simulink model "msgex1_data_vs_event_vs_msg"  (R2018a)
settings: Solver=FixedStepDiscrete  StartTime=0.0  StopTime=10.0  FixedStep=1  RelTol=1e-3  EnableMultiTasking=on
undefined symbols (not defined in the file or in its folder): m, n
settings Model: Creator=The MathWorks, Inc.  LastModifiedBy=Michael Girbino
settings DataIOCC: LimitDataPoints=on  SaveFormat=Array
settings OptimizationCC: ExpressionDepthLimit=2147483647  LifeSpan=1
settings DebuggingCC: UnderspecifiedInitializationDetection=Classic  MergeDetectMultiDrivingBlocksExec=none  SolverPrmCheckMsg=warning  AllowSymbolicDim=off  StateNameClashWarn=warning  SFUnexpectedBacktrackingDiag=warning  SFNoUnconditionalDefaultTransitionDiag=warning  SFExecutionAtInitializationDiag=none
settings HardwareCC: ProdBitPerPointer=32  ProdBitPerSizeT=32  ProdBitPerPtrDiffT=32  ProdLargestAtomicFloat=None  ProdIntDivRoundTo=Undefined  ProdEndianess=Unspecified  ProdWordSize=32  ProdHWDeviceType=32-bit Generic
settings ModelReferenceCC: PropagateSignalLabelsOutOfModel=off
settings SFSimCC: MATLABDynamicMemAlloc=off
settings RTWCC: SystemTargetFile=ert.tlc  TemplateMakefile=ert_default_tmf  Description=Real-Time Workshop Embedded Coder
settings CodeAppCC: IgnoreCustomStorageClasses=off  CustomSymbolStrType=$N$R$M  StateflowObjectComments=on  InternalIdentifier=Classic
settings ERTTargetCC: MultiwordLength=2048  GenerateSampleERTMain=on  ERTCustomFileTemplate=example_file_process.tlc  ConvertIfToSwitch=off  SuppressUnreachableDefaultCases=off
settings ConfigComp: CovMetricSettings=dw  CovHtmlReporting=on  CovSaveCumulativeToWorkspaceVar=on  CovSaveSingleToWorkspaceVar=on  CovExternalEMLEnable=off  CovSFcnEnable=off

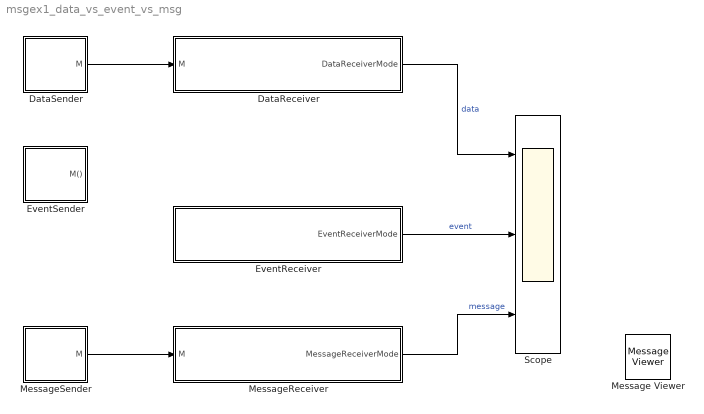
== system msgex1_data_vs_event_vs_msg ==
  DataReceiver : Stateflow chart  TreatAsAtomicUnit=on
  DataSender : Stateflow chart  TreatAsAtomicUnit=on
  EventReceiver : Stateflow chart  TreatAsAtomicUnit=on
  EventSender : Stateflow chart  TreatAsAtomicUnit=on
  Message Viewer : MessageViewer
  MessageReceiver : Stateflow chart  TreatAsAtomicUnit=on
  MessageSender : Stateflow chart  TreatAsAtomicUnit=on
  Scope : Scope  NumInputPorts=3
  wires:
  MessageSender/1(M) -> MessageReceiver/1(M)
  DataSender/1(M) -> DataReceiver/1(M)
  EventReceiver/1(EventReceiverMode) -> Scope/2  "event"
  MessageReceiver/1(MessageReceiverMode) -> Scope/3  "message"
  DataReceiver/1(DataReceiverMode) -> Scope/1  "data"

== stateflow chart msgex1_data_vs_event_vs_msg/MessageSender ==
  state A
    en:
    send(M);
  (default) -> A
  data: M output double

== stateflow chart msgex1_data_vs_event_vs_msg/MessageReceiver ==
  state A0
  state A1
  state A2
  state A3
  (default) -> A0
  A0 -> A1 : after(3,sec)
  A1 -> A2 : M
  A2 -> A3 : M
  data: M input double; MessageReceiverMode output Enum: MessageReceiverModeType

== stateflow chart msgex1_data_vs_event_vs_msg/EventReceiver ==
  state A0
  state A1
    en: send(M, A2);
  state A2
    en: send(M,A3);
  state A3
  (default) -> A0
  A0 -> A1 : after(3,sec)
  A1 -> A2 : M
  A2 -> A3 : M
  data: EventReceiverMode output Enum: EventReceiverModeType
  events: M local FUNCTION_CALL_EVENT

== stateflow chart msgex1_data_vs_event_vs_msg/EventSender ==
  state A
    en: send(M)
  (default) -> A
  events: M output FUNCTION_CALL_EVENT

== stateflow chart msgex1_data_vs_event_vs_msg/DataReceiver ==
  state A0
  state A1
    en: A = 1;
    du: B = 1;
    ex: C = 1;
    state CorrectFalseReversePending
      (default) -> (junction 119)
      (junction 119) -> (junction 115) [order 1] : [true]
      (junction 119) -> (junction 120) [order 2]
      (junction 115) -> (junction 112) : {D = 1;
          | }
      (junction 112) -> (junction 120)
    state CorrectTrueReversePending
      (default) -> (junction 122)
      (junction 122) -> (junction 111) [order 1] : [true]
      (junction 122) -> (junction 110) [order 2]
      (junction 111) -> (junction 121) : {E = 2;}
      (junction 121) -> (junction 110)
    state Finished1
      E = 1;
    (default) -> (junction 118)
    (junction 118) -> CorrectFalseReversePending [order 1] : [true]
    (junction 118) -> (junction 125) [order 2]
    CorrectFalseReversePending -> (junction 125)
    (junction 125) -> (junction 126)
    (junction 126) -> CorrectTrueReversePending [order 1] : [true]
    (junction 126) -> (junction 127) [order 2]
    CorrectTrueReversePending -> (junction 127)
    (junction 127) -> Finished1
  state Finished [commented out]
  state A2
  state A3
  (default) -> A0
  A0 -> A1 : after(3,sec)
  (default) -> (junction 18) [commented out] : {E = 1;}
  (junction 18) -> (junction 15) [commented out] : [true]
  (junction 15) -> (junction 33) [commented out] : {D=1;
      | }
  (junction 18) -> Finished [commented out]
  (junction 33) -> (junction 26) [commented out] : [true]
  (junction 33) -> (junction 34) [commented out]
  (junction 26) -> (junction 29) [commented out] : {D=2;
      | }
  (junction 29) -> (junction 34) [commented out]
  (junction 34) -> (junction 13) [commented out]
  (junction 13) -> Finished [commented out]
  A1 -> A2 : [E == 1]
  A2 -> A3 : [E == 1]
  data: M input double; DataReceiverMode output Enum: DataReceiverModeType; A local; B local; C local; D local; E local =0

== stateflow chart msgex1_data_vs_event_vs_msg/DataSender ==
  state A
    en: M = 1;
  (default) -> A
  data: M output double
